simulink model "parallel_parking"  (R2019b)
settings: Solver=VariableStepAuto  StartTime=0.0  StopTime=20.0  RelTol=1e-3
values from neighbouring files (symbols this model uses):
  delta_max = 20    [Initialize_controller_parameter.m]
  parking_speed = 0.1    [Initialize_controller_parameter.m]
  TOF_distance_limit = 20    [Initialize_controller_parameter.m]
libraries: simulink x4

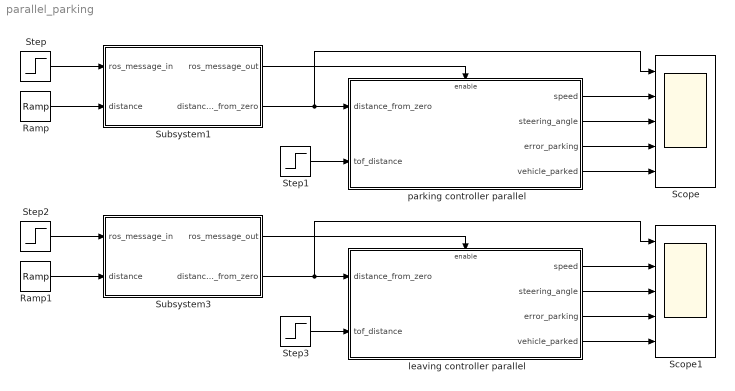
== system parallel_parking ==
  Ramp : simulink/Sources/Ramp  slope=100  start=0  InitialOutput=0
  Ramp1 : simulink/Sources/Ramp  slope=100  start=0  InitialOutput=0
  Scope : Scope  NumInputPorts=5
  Scope1 : Scope  NumInputPorts=5
  Step : Step  Time=2  SampleTime=0
  Step1 : Step  Time=13  Before=30  After=10  SampleTime=0
  Step2 : Step  Time=2  SampleTime=0
  Step3 : Step  Time=13  Before=30  After=10  SampleTime=0
  Subsystem1 : Subsystem
  Subsystem3 : Subsystem
  leaving controller parallel : Subsystem
  parking controller parallel : Subsystem
  wires:
  Subsystem1/2(distance_from_zero) -> Scope/1, parking controller parallel/1(distance_from_zero)
  Subsystem1/1("ros_message_out ") -> parking controller parallel/Enable
  Step/1 -> Subsystem1/1(ros_message_in)
  Ramp/1 -> Subsystem1/2(distance)
  Step1/1 -> parking controller parallel/2(tof_distance)
  parking controller parallel/1(speed) -> Scope/2
  parking controller parallel/2(steering_angle) -> Scope/3
  parking controller parallel/3(error_parking) -> Scope/4
  parking controller parallel/4("vehicle_parked ") -> Scope/5
  leaving controller parallel/3(error_parking) -> Scope1/4
  Subsystem3/1("ros_message_out ") -> leaving controller parallel/Enable
  Step2/1 -> Subsystem3/1(ros_message_in)
  leaving controller parallel/1(speed) -> Scope1/2
  Step3/1 -> leaving controller parallel/2(tof_distance)
  leaving controller parallel/4("vehicle_parked ") -> Scope1/5
  leaving controller parallel/2(steering_angle) -> Scope1/3
  Subsystem3/2(distance_from_zero) -> Scope1/1, leaving controller parallel/1(distance_from_zero)
  Ramp1/1 -> Subsystem3/2(distance)

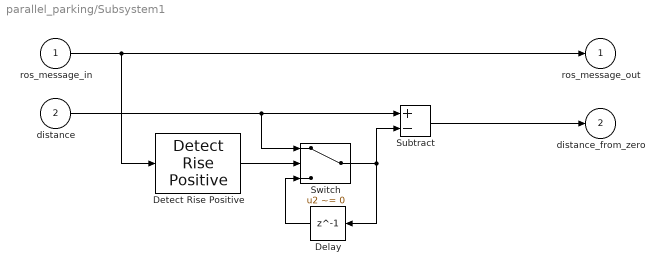
== system parallel_parking/Subsystem1 ==
  ros_message_in : Inport
  distance : Inport  Port=2
  Delay : Delay  DelayLength=1
  "Detect Rise Positive " : simulink/Logic and Bit Operations/Detect Rise Positive  vinit=0  OutDataTypeStr=boolean
  Subtract : Sum  Inputs=+-
  Switch : Switch  Criteria=u2 ~= 0
  "ros_message_out " : Outport
  distance_from_zero : Outport  Port=2
  wires:
  ros_message_in/1 -> "Detect Rise Positive "/1, "ros_message_out "/1
  Delay/1 -> Switch/3
  Subtract/1 -> distance_from_zero/1
  distance/1 -> Switch/1, Subtract/1
  Switch/1 -> Subtract/2, Delay/1
  "Detect Rise Positive "/1 -> Switch/2

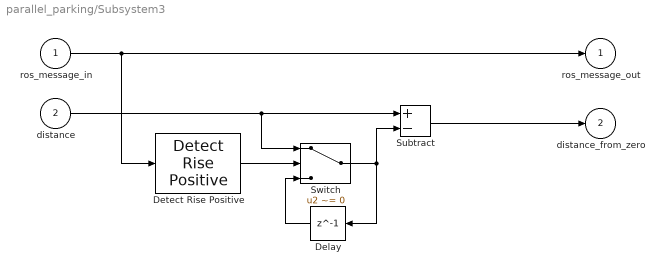
== system parallel_parking/Subsystem3 ==
  ros_message_in : Inport
  distance : Inport  Port=2
  Delay : Delay  DelayLength=1
  "Detect Rise Positive " : simulink/Logic and Bit Operations/Detect Rise Positive  vinit=0  OutDataTypeStr=boolean
  Subtract : Sum  Inputs=+-
  Switch : Switch  Criteria=u2 ~= 0
  "ros_message_out " : Outport
  distance_from_zero : Outport  Port=2
  wires:
  ros_message_in/1 -> "Detect Rise Positive "/1, "ros_message_out "/1
  Delay/1 -> Switch/3
  Subtract/1 -> distance_from_zero/1
  distance/1 -> Switch/1, Subtract/1
  Switch/1 -> Subtract/2, Delay/1
  "Detect Rise Positive "/1 -> Switch/2

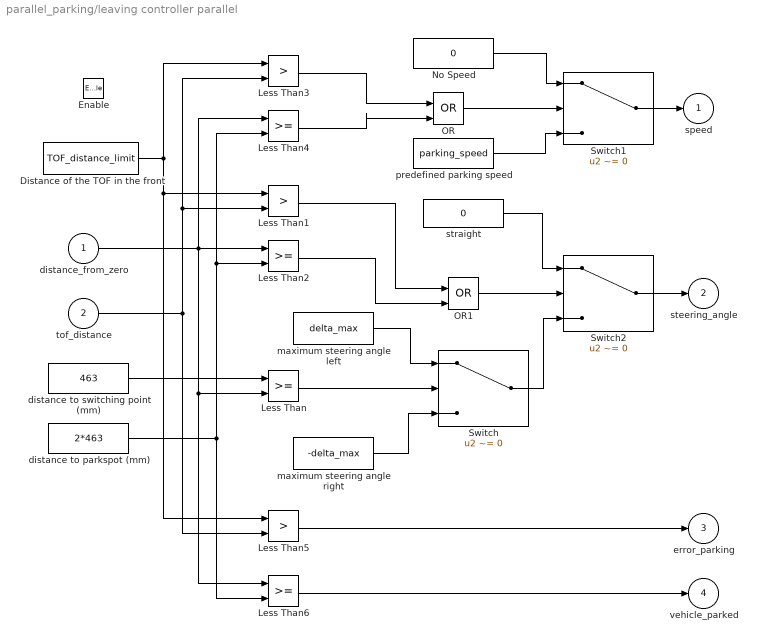
== system parallel_parking/leaving controller parallel ==
  distance_from_zero : Inport
  tof_distance : Inport  Port=2
  Enable : EnablePort
  "Distance of the TOF in the front " : Constant  Value=TOF_distance_limit
  Less Than{,2,4,6} (4 alike) : RelationalOperator  OutDataTypeStr=boolean  RndMeth=Simplest
  Less Than1 : RelationalOperator  Operator=>  OutDataTypeStr=boolean  RndMeth=Simplest
  Less Than3 : RelationalOperator  Operator=>  OutDataTypeStr=boolean  RndMeth=Simplest
  Less Than5 : RelationalOperator  Operator=>  OutDataTypeStr=boolean  RndMeth=Simplest
  No Speed : Constant  Value=0
  OR : Logic  Operator=OR  IconShape=distinctive  AllPortsSameDT=off  OutDataTypeStr=boolean
  OR1 : Logic  Operator=OR  IconShape=distinctive  AllPortsSameDT=off  OutDataTypeStr=boolean
  Switch : Switch  Criteria=u2 ~= 0  Threshold=1079  OutDataTypeStr=single
  Switch1 : Switch  Criteria=u2 ~= 0  Threshold=1377  OutDataTypeStr=single
  Switch2 : Switch  Criteria=u2 ~= 0  Threshold=1079  OutDataTypeStr=single
  distance to parkspot (mm) : Constant  Value=2*463
  "distance to switching point (mm) " : Constant  Value=463
  maximum steering angle left : Constant  Value=delta_max
  maximum steering angle right : Constant  Value=-delta_max
  predefined parking speed : Constant  Value=parking_speed
  straight : Constant  Value=0
  speed : Outport
  steering_angle : Outport  Port=2
  error_parking : Outport  Port=3
  "vehicle_parked " : Outport  Port=4
  wires:
  maximum steering angle right/1 -> Switch/3
  Less Than/1 -> Switch/2
  predefined parking speed/1 -> Switch1/3
  No Speed/1 -> Switch1/1
  Switch/1 -> Switch2/3
  OR/1 -> Switch1/2
  Switch1/1 -> speed/1
  maximum steering angle left/1 -> Switch/1
  Switch2/1 -> steering_angle/1
  straight/1 -> Switch2/1
  "distance to switching point (mm) "/1 -> Less Than/1
  distance_from_zero/1 -> Less Than6/1, Less Than/2, Less Than2/1, Less Than4/1
  OR1/1 -> Switch2/2
  tof_distance/1 -> Less Than5/2, Less Than1/2, Less Than3/2
  "Distance of the TOF in the front "/1 -> Less Than3/1, Less Than5/1, Less Than1/1
  distance to parkspot (mm)/1 -> Less Than4/2, Less Than2/2, Less Than6/2
  Less Than2/1 -> OR1/2
  Less Than1/1 -> OR1/1
  Less Than3/1 -> OR/1
  Less Than4/1 -> OR/2
  Less Than6/1 -> "vehicle_parked "/1
  Less Than5/1 -> error_parking/1

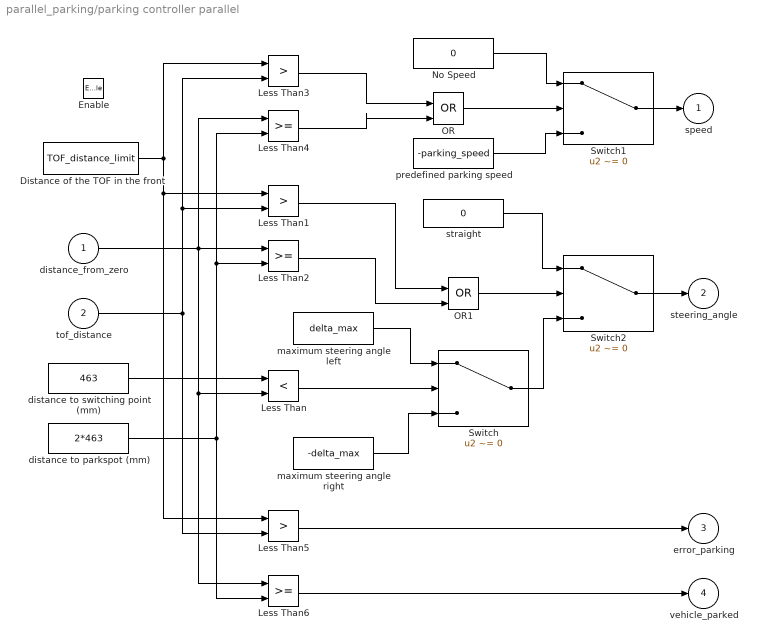
== system parallel_parking/parking controller parallel ==
  distance_from_zero : Inport
  tof_distance : Inport  Port=2
  Enable : EnablePort
  "Distance of the TOF in the front " : Constant  Value=TOF_distance_limit
  Less Than : RelationalOperator  Operator=<  OutDataTypeStr=boolean  RndMeth=Simplest
  Less Than1 : RelationalOperator  Operator=>  OutDataTypeStr=boolean  RndMeth=Simplest
  Less Than2 : RelationalOperator  OutDataTypeStr=boolean  RndMeth=Simplest
  Less Than3 : RelationalOperator  Operator=>  OutDataTypeStr=boolean  RndMeth=Simplest
  Less Than4 : RelationalOperator  OutDataTypeStr=boolean  RndMeth=Simplest
  Less Than5 : RelationalOperator  Operator=>  OutDataTypeStr=boolean  RndMeth=Simplest
  Less Than6 : RelationalOperator  OutDataTypeStr=boolean  RndMeth=Simplest
  No Speed : Constant  Value=0
  OR : Logic  Operator=OR  IconShape=distinctive  AllPortsSameDT=off  OutDataTypeStr=boolean
  OR1 : Logic  Operator=OR  IconShape=distinctive  AllPortsSameDT=off  OutDataTypeStr=boolean
  Switch : Switch  Criteria=u2 ~= 0  Threshold=1079  OutDataTypeStr=single
  Switch1 : Switch  Criteria=u2 ~= 0  Threshold=1377  OutDataTypeStr=single
  Switch2 : Switch  Criteria=u2 ~= 0  Threshold=1079  OutDataTypeStr=single
  distance to parkspot (mm) : Constant  Value=2*463
  "distance to switching point (mm) " : Constant  Value=463
  maximum steering angle left : Constant  Value=delta_max
  maximum steering angle right : Constant  Value=-delta_max
  predefined parking speed : Constant  Value=-parking_speed
  straight : Constant  Value=0
  speed : Outport
  steering_angle : Outport  Port=2
  error_parking : Outport  Port=3
  "vehicle_parked " : Outport  Port=4
  wires:
  maximum steering angle right/1 -> Switch/3
  Less Than/1 -> Switch/2
  predefined parking speed/1 -> Switch1/3
  No Speed/1 -> Switch1/1
  Switch/1 -> Switch2/3
  OR/1 -> Switch1/2
  Switch1/1 -> speed/1
  maximum steering angle left/1 -> Switch/1
  Switch2/1 -> steering_angle/1
  straight/1 -> Switch2/1
  "distance to switching point (mm) "/1 -> Less Than/1
  distance_from_zero/1 -> Less Than6/1, Less Than/2, Less Than2/1, Less Than4/1
  OR1/1 -> Switch2/2
  tof_distance/1 -> Less Than5/2, Less Than1/2, Less Than3/2
  "Distance of the TOF in the front "/1 -> Less Than3/1, Less Than5/1, Less Than1/1
  distance to parkspot (mm)/1 -> Less Than4/2, Less Than2/2, Less Than6/2
  Less Than2/1 -> OR1/2
  Less Than1/1 -> OR1/1
  Less Than3/1 -> OR/1
  Less Than4/1 -> OR/2
  Less Than6/1 -> "vehicle_parked "/1
  Less Than5/1 -> error_parking/1
